simulink model "Example"  (R2019b)
settings: Solver=VariableStepAuto  StartTime=0.0  StopTime=100  RelTol=1e-3
libraries: ForceSeatDI_Simulink x2
settings Model: EnablePacing=on  Creator=usr  LastModifiedBy=usr

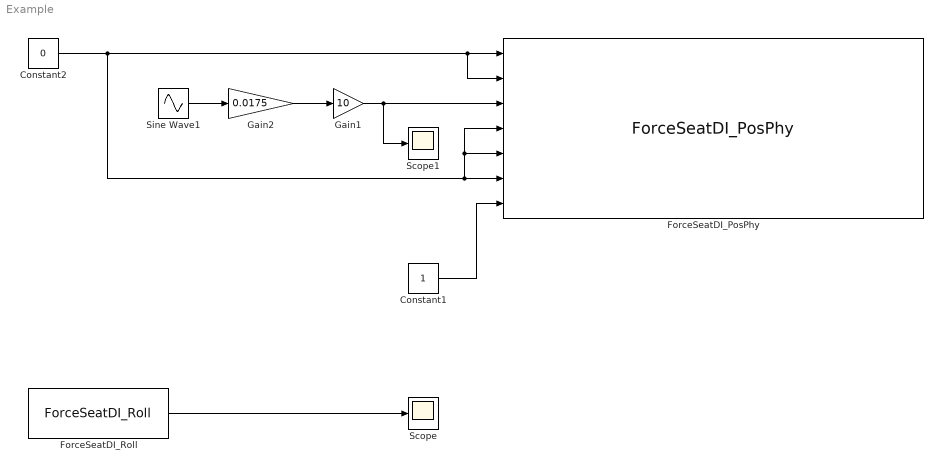
== system Example ==
  Constant1 : Constant  OutDataTypeStr=int32
  Constant2 : Constant  Value=0
  ForceSeatDI_PosPhy : ForceSeatDI_Simulink/ForceSeatDI_PosPhy
      settings: SourceProductName=MotionsSystems ForceSeatDI
  ForceSeatDI_Roll : ForceSeatDI_Simulink/ForceSeatDI_Roll
      settings: SourceProductName=MotionsSystems ForceSeatDI
  Gain1 : Gain  Gain=10
  Gain2 : Gain  Gain=0.0175
  Scope : Scope
  Scope1 : Scope
  Sine Wave1 : Sin  SampleTime=0.01
  wires:
  Constant1/1 -> ForceSeatDI_PosPhy/7
  Constant2/1 -> ForceSeatDI_PosPhy/1, ForceSeatDI_PosPhy/2, ForceSeatDI_PosPhy/6, ForceSeatDI_PosPhy/5, ForceSeatDI_PosPhy/4
  Sine Wave1/1 -> Gain2/1
  Gain2/1 -> Gain1/1
  Gain1/1 -> ForceSeatDI_PosPhy/3, Scope1/1
  ForceSeatDI_Roll/1 -> Scope/1
